simulink model "Balanced_Infantry"  (R2020a)
settings: Solver=FixedStepDiscrete  StartTime=0.0  StopTime=inf  FixedStep=0.001  RelTol=1e-3
model workspace (MAT data in the model file):
  L_K = 1
  L_pressure = 1
  L_rebound = 1
  R_K = 1
libraries: STM32_Config_Lib x1
settings Model: Creator=ly  LastModifiedBy=hall
settings OptimizationCC: DefaultParameterBehavior=Inlined  EnhancedBackFolding=on  PassReuseOutputArgsAs=Individual arguments  ZeroExternalMemoryAtStartup=off  ZeroInternalMemoryAtStartup=off  OptimizeBlockOrder=speed  DifferentSizesBufferReuse=on  OptimizationCustomize=off  EfficientTunableParamExpr=on
settings DebuggingCC: ParameterTunabilityLossMsg=error
settings HardwareCC: ProdBitPerPointer=32  ProdBitPerSizeT=32  ProdBitPerPtrDiffT=32  ProdLargestAtomicInteger=Long  ProdWordSize=32  ProdHWDeviceType=STM32CortexM
settings SFSimCC: MATLABDynamicMemAlloc=off
settings RTWCC: Description=stm32 (Embedded Target)  SystemTargetFile=stm32.tlc  TemplateMakefile=stm32.tmf  GenerateReport=on
settings CodeAppCC: ForceParamTrailComments=on  IgnoreCustomStorageClasses=off  MaxIdLength=64  OperatorAnnotations=on  SimulinkDataObjDesc=on  SFDataObjDesc=on  CustomSymbolStrType=$N$R$M  SimulinkBlockComments=off
settings STFCustomTargetCC: TargetLangStandard=C99 (ISO)  CodeReplacementLibrary=ARM CMSIS SIN COS  MultiwordLength=256  ParMdlRefBuildCompliant=on  IncludeMdlTerminateFcn=off  CombineOutputUpdateFcns=on  ERTCustomFileBanners=on  SupportContinuousTime=off  SupportNonInlinedSFcns=off  RemoveResetFunc=on  MATLABClassNameForMDSCustomization=Simulink.SoftwareTarget.ERTCustomization  SystemTargetFile=stm32.tlc
settings ERTTargetCC: TargetLangStandard=C99 (ISO)  CodeReplacementLibrary=ARM CMSIS SIN COS  CompOptLevelCompliant=off  ConcurrentExecutionCompliant=off  IncludeMdlTerminateFcn=off  ModelStepFunctionPrototypeControlCompliant=off  CPPClassGenCompliant=off  UseToolchainInfoCompliant=off  ExtModeStaticAllocSize=256  ExtModeMexFile=ext_serial_win32_comm  ExtModeMexArgs=0,1,115200,10  InlinedParameterPlacement=NonHierarchical  ERTSrcFileBannerTemplate=sourceFileTemplate.cgt  ERTHdrFileBannerTemplate=sourceFileTemplate.cgt  ERTDataSrcFileTemplate=sourceFileTemplate.cgt  ERTDataHdrFileTemplate=sourceFileTemplate.cgt  ERTCustomFileTemplate=customRoutineProcess.tlc

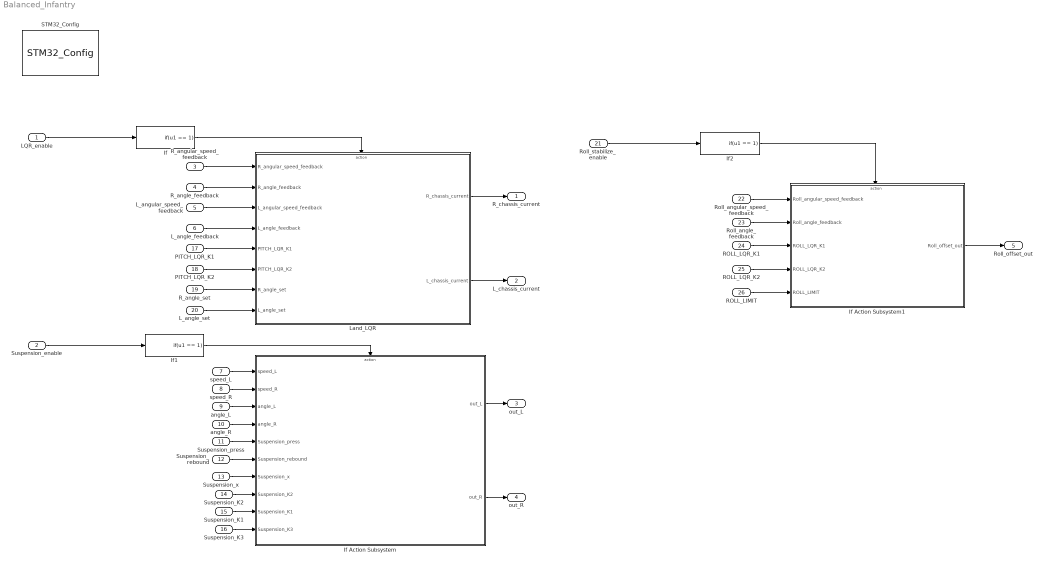
== system Balanced_Infantry ==
  LQR_enable : Inport
  Suspension_enable : Inport  Port=2
  R_angular_speed_feedback : Inport  Port=3
  R_angle_feedback : Inport  Port=4
  L_angular_speed_feedback : Inport  Port=5
  L_angle_feedback : Inport  Port=6
  speed_L : Inport  Port=7
  speed_R : Inport  Port=8
  angle_L : Inport  Port=9
  angle_R : Inport  Port=10
  Suspension_press : Inport  Port=11
  Suspension_rebound : Inport  Port=12
  Suspension_x : Inport  Port=13
  Suspension_K2 : Inport  Port=14
  Suspension_K1 : Inport  Port=15
  Suspension_K3 : Inport  Port=16
  PITCH_LQR_K1 : Inport  Port=17
  PITCH_LQR_K2 : Inport  Port=18
  R_angle_set : Inport  Port=19
  L_angle_set : Inport  Port=20
  Roll_stabilize_enable : Inport  Port=21
  Roll_angular_speed_feedback : Inport  Port=22
  Roll_angle_feedback : Inport  Port=23
  ROLL_LQR_K1 : Inport  Port=24
  ROLL_LQR_K2 : Inport  Port=25
  ROLL_LIMIT : Inport  Port=26
  If : If  IfExpression=u1 == 1  ShowElse=off
  If Action Subsystem : Subsystem  TreatAsAtomicUnit=on
  If Action Subsystem1 : Subsystem  TreatAsAtomicUnit=on
  If1 : If  IfExpression=u1 == 1  ShowElse=off
  If2 : If  IfExpression=u1 == 1  ShowElse=off
  Land_LQR : Subsystem  TreatAsAtomicUnit=on
  STM32_Config : STM32_Config_Lib/STM32_Config  Priority=0  Project_Path=.\  Config_File=Balanced_Infantry.ioc  MCU_Name=STM32F407IGHx
      settings: SourceProductName=Target Support Package - STM32 Adapter
  R_chassis_current : Outport
  L_chassis_current : Outport  Port=2
  out_L : Outport  Port=3
  out_R : Outport  Port=4
  Roll_offset_out : Outport  Port=5
  wires:
  If/1 -> Land_LQR/Action
  If1/1 -> If Action Subsystem/Action
  Land_LQR/1(R_chassis_current) -> R_chassis_current/1
  Land_LQR/2(L_chassis_current) -> L_chassis_current/1
  R_angular_speed_feedback/1 -> Land_LQR/1(R_angular_speed_feedback)
  R_angle_feedback/1 -> Land_LQR/2(R_angle_feedback)
  L_angular_speed_feedback/1 -> Land_LQR/3(L_angular_speed_feedback)
  L_angle_feedback/1 -> Land_LQR/4(L_angle_feedback)
  speed_L/1 -> If Action Subsystem/1(speed_L)
  speed_R/1 -> If Action Subsystem/2(speed_R)
  angle_L/1 -> If Action Subsystem/3(angle_L)
  angle_R/1 -> If Action Subsystem/4(angle_R)
  If Action Subsystem/1(out_L) -> out_L/1
  If Action Subsystem/2(out_R) -> out_R/1
  Suspension_press/1 -> If Action Subsystem/5(Suspension_press)
  Suspension_rebound/1 -> If Action Subsystem/6(Suspension_rebound)
  Suspension_x/1 -> If Action Subsystem/7(Suspension_x)
  Suspension_K2/1 -> If Action Subsystem/8(Suspension_K2)
  Suspension_K1/1 -> If Action Subsystem/9(Suspension_K1)
  Suspension_K3/1 -> If Action Subsystem/10(Suspension_K3)
  LQR_enable/1 -> If/1
  Suspension_enable/1 -> If1/1
  PITCH_LQR_K1/1 -> Land_LQR/5(PITCH_LQR_K1)
  PITCH_LQR_K2/1 -> Land_LQR/6(PITCH_LQR_K2)
  R_angle_set/1 -> Land_LQR/7(R_angle_set)
  L_angle_set/1 -> Land_LQR/8(L_angle_set)
  Roll_stabilize_enable/1 -> If2/1
  If2/1 -> If Action Subsystem1/Action
  Roll_angular_speed_feedback/1 -> If Action Subsystem1/1(Roll_angular_speed_feedback)
  Roll_angle_feedback/1 -> If Action Subsystem1/2(Roll_angle_feedback)
  ROLL_LQR_K1/1 -> If Action Subsystem1/3(ROLL_LQR_K1)
  ROLL_LQR_K2/1 -> If Action Subsystem1/4(ROLL_LQR_K2)
  If Action Subsystem1/1(Roll_offset_out) -> Roll_offset_out/1
  ROLL_LIMIT/1 -> If Action Subsystem1/5(ROLL_LIMIT)

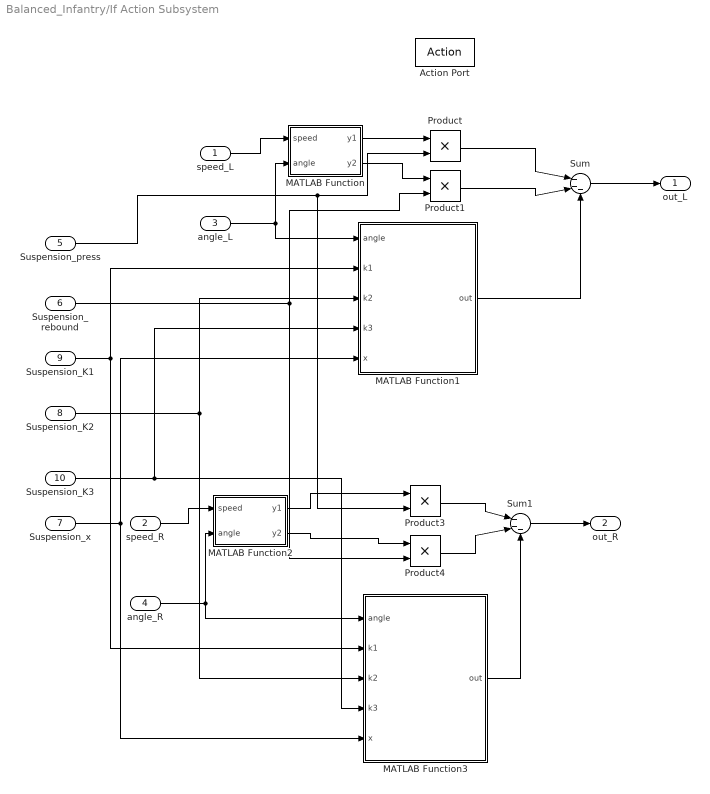
== system Balanced_Infantry/If Action Subsystem ==
  speed_L : Inport
  speed_R : Inport  Port=2
  angle_L : Inport  Port=3
  angle_R : Inport  Port=4
  Suspension_press : Inport  Port=5
  Suspension_rebound : Inport  Port=6
  Suspension_x : Inport  Port=7
  Suspension_K2 : Inport  Port=8
  Suspension_K1 : Inport  Port=9
  Suspension_K3 : Inport  Port=10
  Action Port : ActionPort  ActionPortLabel=if(u1 == 1)
  MATLAB Function : MATLAB Function  TreatAsAtomicUnit=on
  MATLAB Function1 : MATLAB Function  TreatAsAtomicUnit=on
  MATLAB Function2 : MATLAB Function  TreatAsAtomicUnit=on
  MATLAB Function3 : MATLAB Function  TreatAsAtomicUnit=on
  Product{,1,3..4} (4 alike) : Product
  Sum : Sum  Inputs=|---
  Sum1 : Sum  Inputs=|---
  out_L : Outport
  out_R : Outport  Port=2
  wires:
  Sum/1 -> out_L/1
  Product/1 -> Sum/1
  Sum1/1 -> out_R/1
  angle_L/1 -> MATLAB Function/2(angle), MATLAB Function1/1(angle)
  angle_R/1 -> MATLAB Function2/2(angle), MATLAB Function3/1(angle)
  speed_L/1 -> MATLAB Function/1(speed)
  MATLAB Function/1(y1) -> Product/1
  MATLAB Function/2(y2) -> Product1/1
  Product1/1 -> Sum/2
  speed_R/1 -> MATLAB Function2/1(speed)
  MATLAB Function2/1(y1) -> Product3/1
  MATLAB Function2/2(y2) -> Product4/1
  Product3/1 -> Sum1/1
  Product4/1 -> Sum1/2
  Suspension_press/1 -> Product/2, Product3/2
  Suspension_rebound/1 -> Product1/2, Product4/2
  Suspension_K1/1 -> MATLAB Function1/2(k1), MATLAB Function3/2(k1)
  MATLAB Function1/1(out) -> Sum/3
  Suspension_K2/1 -> MATLAB Function3/3(k2), MATLAB Function1/3(k2)
  Suspension_K3/1 -> MATLAB Function3/4(k3), MATLAB Function1/4(k3)
  Suspension_x/1 -> MATLAB Function3/5(x), MATLAB Function1/5(x)
  MATLAB Function3/1(out) -> Sum1/3

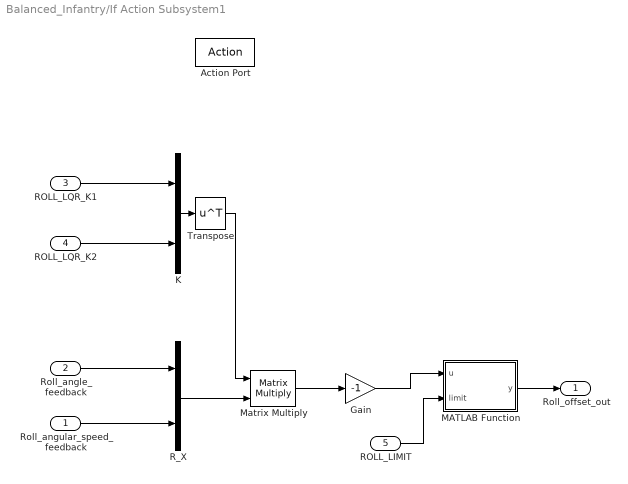
== system Balanced_Infantry/If Action Subsystem1 ==
  Roll_angular_speed_feedback : Inport
  Roll_angle_feedback : Inport  Port=2
  ROLL_LQR_K1 : Inport  Port=3
  ROLL_LQR_K2 : Inport  Port=4
  ROLL_LIMIT : Inport  Port=5
  Action Port : ActionPort  ActionPortLabel=if(u1 == 1)
  Gain : Gain  Gain=-1
  K : Mux  Inputs=2
  MATLAB Function : MATLAB Function  TreatAsAtomicUnit=on
  Matrix Multiply : Product  Multiplication=Matrix(*)
  R_X : Mux  Inputs=2
  Transpose : Math  Operator=transpose  SaturateOnIntegerOverflow=on
  Roll_offset_out : Outport
  wires:
  Roll_angular_speed_feedback/1 -> R_X/2
  Roll_angle_feedback/1 -> R_X/1
  Transpose/1 -> Matrix Multiply/1
  K/1 -> Transpose/1
  Matrix Multiply/1 -> Gain/1
  R_X/1 -> Matrix Multiply/2
  ROLL_LQR_K1/1 -> K/1
  ROLL_LQR_K2/1 -> K/2
  Gain/1 -> MATLAB Function/1(u)
  MATLAB Function/1(y) -> Roll_offset_out/1
  ROLL_LIMIT/1 -> MATLAB Function/2(limit)

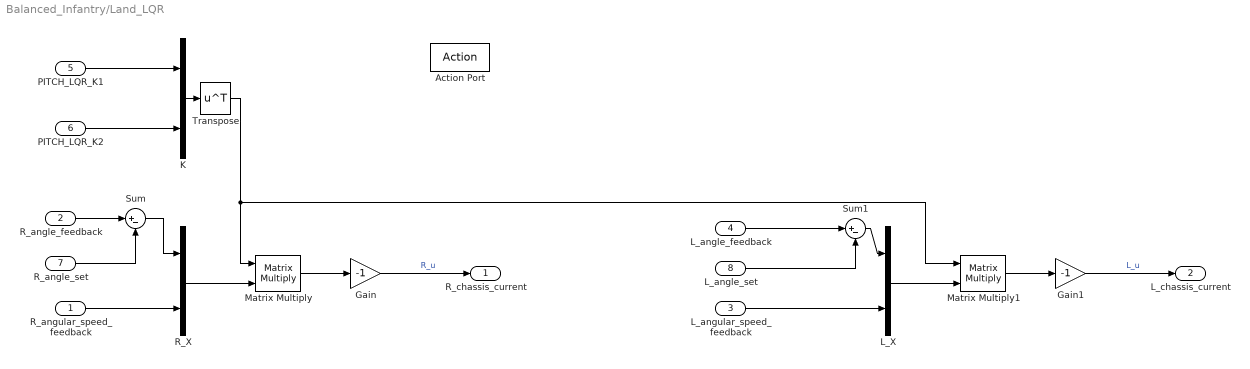
== system Balanced_Infantry/Land_LQR ==
  R_angular_speed_feedback : Inport
  R_angle_feedback : Inport  Port=2
  L_angular_speed_feedback : Inport  Port=3
  L_angle_feedback : Inport  Port=4
  PITCH_LQR_K1 : Inport  Port=5
  PITCH_LQR_K2 : Inport  Port=6
  R_angle_set : Inport  Port=7
  L_angle_set : Inport  Port=8
  Action Port : ActionPort  ActionPortLabel=if(u1 == 1)
  Gain : Gain  Gain=-1
  Gain1 : Gain  Gain=-1
  K : Mux  Inputs=2
  L_X : Mux  Inputs=2
  Matrix Multiply : Product  Multiplication=Matrix(*)
  Matrix Multiply1 : Product  Multiplication=Matrix(*)
  R_X : Mux  Inputs=2
  Sum : Sum  Inputs=|+-
  Sum1 : Sum  Inputs=|+-
  Transpose : Math  Operator=transpose  SaturateOnIntegerOverflow=on
  R_chassis_current : Outport
  L_chassis_current : Outport  Port=2
  wires:
  PITCH_LQR_K1/1 -> K/1
  PITCH_LQR_K2/1 -> K/2
  R_angular_speed_feedback/1 -> R_X/2
  R_X/1 -> Matrix Multiply/2
  Matrix Multiply/1 -> Gain/1
  Gain/1 -> R_chassis_current/1  "R_u"
  L_X/1 -> Matrix Multiply1/2
  Gain1/1 -> L_chassis_current/1  "L_u"
  L_angular_speed_feedback/1 -> L_X/2
  Matrix Multiply1/1 -> Gain1/1
  K/1 -> Transpose/1
  Transpose/1 -> Matrix Multiply/1, Matrix Multiply1/1
  Sum/1 -> R_X/1
  R_angle_feedback/1 -> Sum/1
  R_angle_set/1 -> Sum/2
  Sum1/1 -> L_X/1
  L_angle_feedback/1 -> Sum1/1
  L_angle_set/1 -> Sum1/2

== matlab function Balanced_Infantry/If Action Subsystem/MATLAB Function1 ==
  data: angle input; out output; k1 input; k2 input; k3 input; x input
function out = fcn(angle,k1,k2,k3,x)
out=0;
if(angle>0&&angle<x)
    out = angle*k1;
elseif (angle<=0)
    out = angle*k3;
elseif (angle>=x)
    out = (angle-x)*k2+k1*x;
end

== matlab function Balanced_Infantry/If Action Subsystem/MATLAB Function ==
  data: speed input; y1 output; y2 output; angle input
function [y1,y2]= fcn(speed,angle)
y1=0;
y2=0;
if(speed*angle>0)
    y1 = speed;
    y2 = 0;
else
    y2 = speed;
    y1 = 0;
end

== matlab function Balanced_Infantry/If Action Subsystem/MATLAB Function2 ==
  data: speed input; y1 output; y2 output; angle input
function [y1,y2]= fcn(speed,angle)
y1=0;
y2=0;
if(speed*angle>0)
    y1 = speed;
    y2 = 0;
else
    y2 = speed;
    y1 = 0;
end

== matlab function Balanced_Infantry/If Action Subsystem/MATLAB Function3 ==
  data: angle input; out output; k1 input; k2 input; k3 input; x input
function out = fcn(angle,k1,k2,k3,x)
out=0;
if(angle>0&&angle<x)
    out = angle*k1;
elseif (angle<=0)
    out = angle*k3;
elseif (angle>=x)
    out = (angle-x)*k2+k1*x;
end

== matlab function Balanced_Infantry/If Action Subsystem1/MATLAB Function ==
  data: u input; y output; limit input
function y = fcn(u,limit)
y=0;
if(abs(u)<=limit)
y = u;
elseif(u>limit)
y=limit;
elseif(u<-limit)
y=-limit;
end
